simulink model "shuzitioapin"  (Simulink 5.0)
settings: Solver=ode45  StartTime=0.0  StopTime=10.0  RelTol=1e-3
libraries: dsparch4 x4, commchan2 x1, commrandsrc2 x1, commsink2 x1, simulink x1, dspsigops x1
settings Model: LastModifiedBy=lenovo

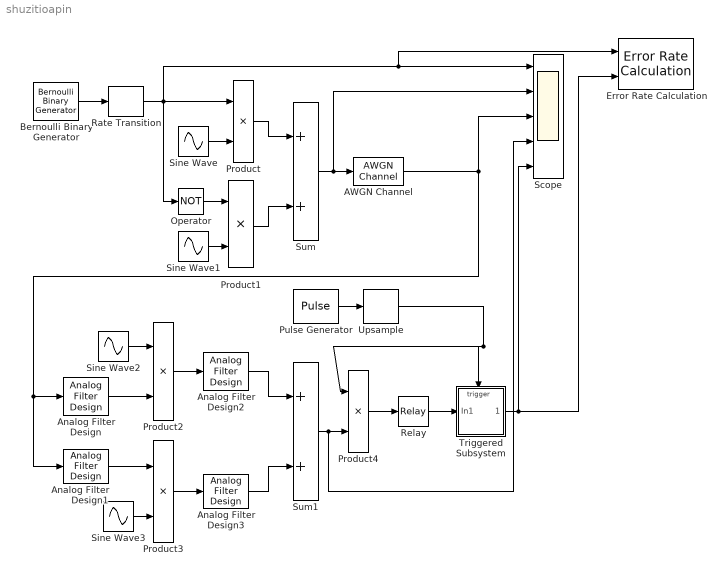
== system shuzitioapin ==
  AWGN Channel : commchan2/AWGN Channel  seed=67  noiseMode=Variance from mask  EsNodB=10  SNRdB=10  Ps=1  Tsym=1  variance=0.5
  Analog Filter Design : dsparch4/Analog Filter Design  method=Butterworth  filttype=Bandpass  N=2  Wlo=2*pi*(100-2)  Whi=2*pi*(100+2)  Rp=2  Rs=40
  Analog Filter Design1 : dsparch4/Analog Filter Design  method=Butterworth  filttype=Bandpass  N=8  Wlo=2*pi*(2000-2)  Whi=2*pi*(2000+2)  Rp=2  Rs=40
  Analog Filter Design2 : dsparch4/Analog Filter Design  method=Butterworth  filttype=Lowpass  N=2  Wlo=2*pi*3  Whi=80  Rp=2  Rs=40
  Analog Filter Design3 : dsparch4/Analog Filter Design  method=Butterworth  filttype=Lowpass  N=2  Wlo=2*pi*3  Whi=80  Rp=2  Rs=40
  Bernoulli Binary Generator : commrandsrc2/Bernoulli Binary Generator  P=0.5  seed=61  Ts=1  frameBased=off  sampPerFrame=1  orient=off
  Error Rate Calculation : commsink2/Error Rate Calculation  N=0  st_delay=0  cp_mode=Entire frame  subframe=[]  PMode=Workspace  WsName=ErrorVec  RsMode2=off  stop=off  numErr=100  maxBits=1e6
  Operator : Logic  Operator=NOT  AllPortsSameDT=off
  Product{,1..4} (5 alike) : Product  SaturateOnIntegerOverflow=on
  Pulse Generator : DiscretePulseGenerator  Period=10  PulseWidth=5  SampleTime=0.1
  Rate Transition : simulink/Signal Attributes/Rate Transition  DataIntegrity=on  DeterministicTransfer=off  TransitionType=Slow to fast  InitCond=0
  Relay : Relay  OnSwitchValue=0.5  OffSwitchValue=0.5
  Scope : Scope  NumInputPorts=5
      settings: YMin=-5~-5~-5~-5~-5  YMax=5~5~5~5~5
  Sine Wave : Sin  Frequency=2*pi*100  SampleTime=0.1
  Sine Wave1 : Sin  Frequency=2*pi*2000  SampleTime=0.1
  Sine Wave2 : Sin  Frequency=2*pi*100  SampleTime=0.1
  Sine Wave3 : Sin  Frequency=2*pi*2000  SampleTime=0.1
  Sum : Sum  SaturateOnIntegerOverflow=on
  Sum1 : Sum  SaturateOnIntegerOverflow=on
  Triggered Subsystem : Subsystem  TreatAsAtomicUnit=on
  Upsample : dspsigops/Upsample  N=10  phase=0  ic=0  mode=Maintain input frame size
  wires:
  Sine Wave/1 -> Product/2
  Rate Transition/1 -> Product/1, Scope/1, Error Rate Calculation/1, Operator/1
  Bernoulli Binary Generator/1 -> Rate Transition/1
  Operator/1 -> Product1/1
  Sine Wave1/1 -> Product1/2
  Product/1 -> Sum/1
  Product1/1 -> Sum/2
  Sum/1 -> AWGN Channel/1, Scope/2
  Analog Filter Design1/1 -> Product3/1
  Sine Wave3/1 -> Product3/2
  Analog Filter Design/1 -> Product2/2
  Sine Wave2/1 -> Product2/1
  Product3/1 -> Analog Filter Design3/1
  Product2/1 -> Analog Filter Design2/1
  Analog Filter Design2/1 -> Sum1/1
  Analog Filter Design3/1 -> Sum1/2
  Product4/1 -> Relay/1
  Pulse Generator/1 -> Upsample/1
  Relay/1 -> Triggered Subsystem/1(In1)
  Sum1/1 -> Product4/2, Scope/4
  Upsample/1 -> Triggered Subsystem/Trigger, Product4/1
  AWGN Channel/1 -> Analog Filter Design1/1, Analog Filter Design/1, Scope/3
  Triggered Subsystem/1(Out1) -> Error Rate Calculation/2, Scope/5

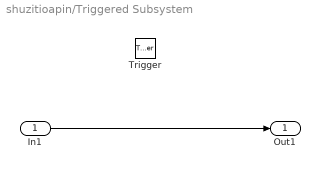
== system shuzitioapin/Triggered Subsystem ==
  In1 : Inport
  Trigger : TriggerPort
  Out1 : Outport
  wires:
  In1/1 -> Out1/1
